simulink library "Thermal_Capacity"  (R2016b)
settings: Solver=ode45  StartTime=0.0  StopTime=10.0  RelTol=1e-3  EnableMultiTasking=on
settings Model: Creator=drhf  LastModifiedBy=drhf
settings DataIOCC: LimitDataPoints=on  SaveFormat=Array  SignalLoggingSaveFormat=ModelDataLogs
settings OptimizationCC: ExpressionDepthLimit=2147483647  LifeSpan=inf
settings DebuggingCC: UnderspecifiedInitializationDetection=Classic  MergeDetectMultiDrivingBlocksExec=none  SolverPrmCheckMsg=warning  FcnCallInpInsideContextMsg=warning  StateNameClashWarn=warning  SFUnexpectedBacktrackingDiag=warning  SFNoUnconditionalDefaultTransitionDiag=warning  SFExecutionAtInitializationDiag=none
settings HardwareCC: ProdBitPerPointer=32  ProdBitPerSizeT=32  ProdBitPerPtrDiffT=32  ProdLargestAtomicFloat=None  ProdIntDivRoundTo=Undefined  ProdEndianess=Unspecified  ProdWordSize=32  ProdHWDeviceType=32-bit Generic
settings ModelReferenceCC: PropagateSignalLabelsOutOfModel=off
settings GRTTargetCC: TargetLangStandard=C89/C90 (ANSI)  GeneratePreprocessorConditionals=Disable all  CombineOutputUpdateFcns=off  GRTInterface=on
settings ConfigComp: CovMetricSettings=dw  CovHtmlReporting=on  CovSaveCumulativeToWorkspaceVar=on  CovSaveSingleToWorkspaceVar=on  CovExternalEMLEnable=off

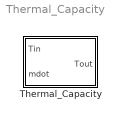
== system Thermal_Capacity ==
  Thermal_Capacity : Subsystem  mask(Thermal Capacity){UA=1, mcp=5*4000, Tamb=20, cp_approx=4200}
      mask prompts: UA "Loss coefficient in W/K"; mcp "Thermal capacity in J/K"; Tamb "Ambient temperature in °C"; cp_approx "heat capacity of fluid in J/kg/K (approximate value)"
      mask help: Basic one node model of a thermal mass using the differential equation:
      mask Help: web(fullfile(path_carnot('help'),'Thermal_Capacity.html'),'-helpbrowser')
      mask TypeOptions UA: Losses/Gain
      mask TypeOptions mcp: Constant/Value
      mask TypeOptions Tamb: Tamb/Value | Integrator/InitialCondition
      mask TypeOptions cp_approx: cp_approx/Value

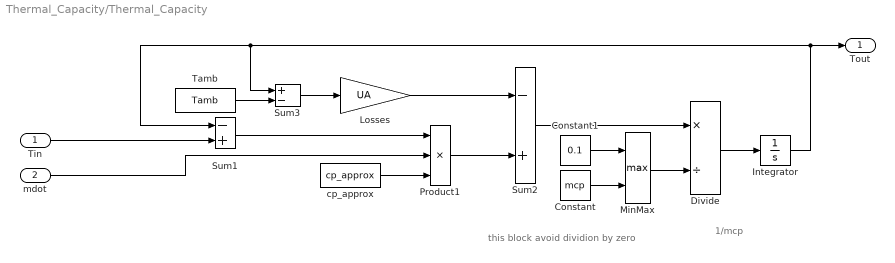
== system Thermal_Capacity/Thermal_Capacity ==
  note: this block avoid dividion by zero
  note: 1/mcp
  Tin : Inport
  mdot : Inport  Port=2
  Constant : Constant  Value=mcp
  Constant1 : Constant  Value=0.1
  Divide : Product  Inputs=*/
  Integrator : Integrator  InitialCondition=Tamb
  Losses : Gain  Gain=UA  SaturateOnIntegerOverflow=on  OutDataTypeStr=Inherit: Same as input  ParamDataTypeStr=Inherit: Same as input
  MinMax : MinMax  Function=max  Inputs=2
  Product1 : Product  Inputs=3  SaturateOnIntegerOverflow=on  InputSameDT=on  OutDataTypeStr=Inherit: Same as first input
  Sum1 : Sum  Inputs=-+  SaturateOnIntegerOverflow=on  InputSameDT=on  OutDataTypeStr=Inherit: Same as first input
  Sum2 : Sum  Inputs=-+  SaturateOnIntegerOverflow=on  InputSameDT=on  OutDataTypeStr=Inherit: Same as first input
  Sum3 : Sum  Inputs=+-  SaturateOnIntegerOverflow=on  InputSameDT=on  OutDataTypeStr=Inherit: Same as first input
  Tamb : Constant  Value=Tamb
  cp_approx : Constant  Value=cp_approx
  Tout : Outport
  wires:
  Constant/1 -> MinMax/2
  Constant1/1 -> MinMax/1
  MinMax/1 -> Divide/2
  mdot/1 -> Product1/2
  Tin/1 -> Sum1/2
  Integrator/1 -> Sum1/1, Sum3/1, Tout/1
  Product1/1 -> Sum2/2
  Sum2/1 -> Divide/1
  Tamb/1 -> Sum3/2
  Losses/1 -> Sum2/1
  Sum3/1 -> Losses/1
  cp_approx/1 -> Product1/3
  Divide/1 -> Integrator/1
  Sum1/1 -> Product1/1
